simulink model "pendulum_2"  (R2023b)
settings: Solver=VariableStepAuto  StartTime=0.0  StopTime=5  RelTol=1e-3
values from neighbouring files (symbols this model uses):
  A = [0   1 ... (first row only)    [DC_motor_example_LQR_v2.m]    (also in inverted_pendulum_main.m = [ 0         0               1                   0)
  Ad = sysd.A    [inverted_pendulum_main.m]
  B = [0 ... (first row only)    [DC_motor_example_LQR_v2.m]    (also in inverted_pendulum_main.m = [       0)
  Bd = sysd.B    [inverted_pendulum_main.m]
  Cc = eye(4)    [inverted_pendulum_main.m]
  Cd = sysd.C    [inverted_pendulum_main.m]
  Dc = zeros(4, 1)    [inverted_pendulum_main.m]
  Dd = sysd.D    [inverted_pendulum_main.m]
  K = lqr(A,B,Q,R)    [DC_motor_example_LQR_v2.m]    (also in inverted_pendulum_main.m = lqr(sys, Qf, Rf))
  Kd = lqr(sysd, Qf, Rf)    [inverted_pendulum_main.m]
  Ts = 0.005    [inverted_pendulum_main.m]
  wc = pi    (= 3.14159265359)    [inverted_pendulum_main.m]
libraries: simulink x8
settings Model: Creator=loicdewit  LastModifiedBy=loicdewit

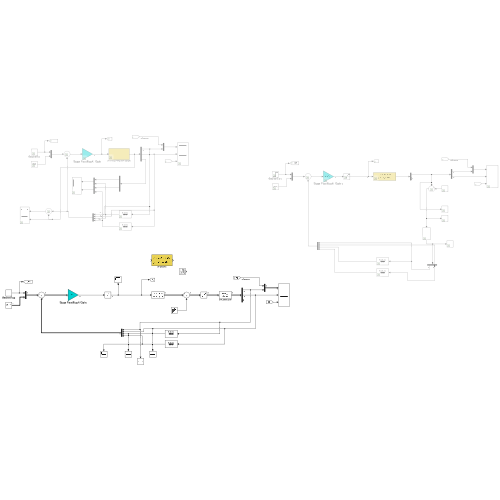
[thumbnail: Simulink's stored preview of the top-level diagram]
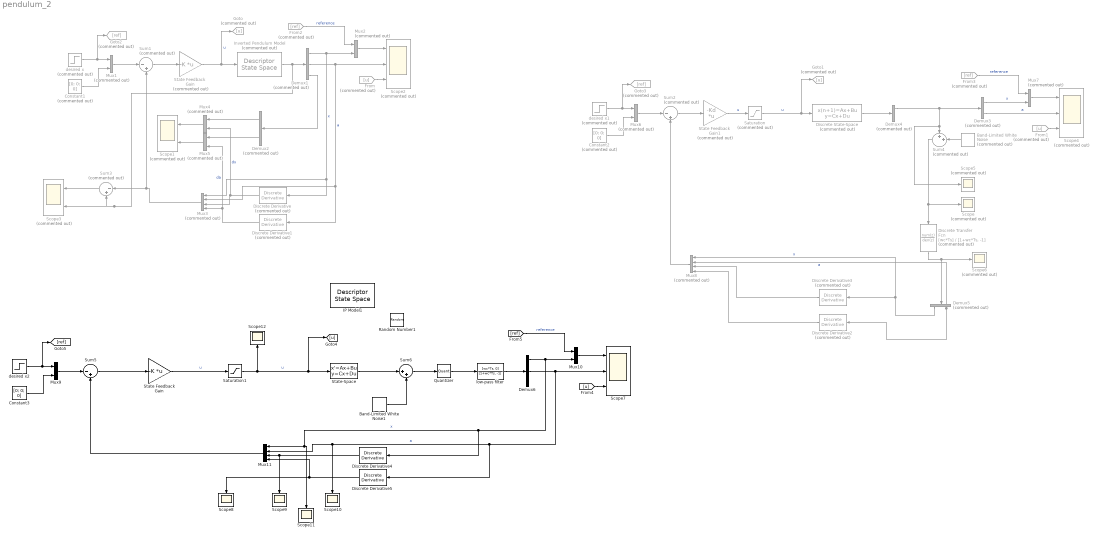
== system pendulum_2 ==
  Band-Limited White Noise : simulink/Sources/Band-Limited White Noise  Commented=on  Cov=[0.000001 * Ts]  Ts=Ts  seed=[13072002]  VectorParams1D=off
  Band-Limited White Noise1 : simulink/Sources/Band-Limited White Noise  Cov=[0.0001 * Ts]  Ts=Ts  seed=[13072002]  VectorParams1D=off
  Constant1 : Constant  Commented=on  Value=[0; 0; 0]
  Constant2 : Constant  Commented=on  Value=[0; 0; 0]
  Constant3 : Constant  Value=[0; 0; 0]  SampleTime=Ts
  Demux1 : Demux  Commented=on  Outputs=[1 1 2]
  Demux2 : Demux  Commented=on  Outputs=[1 1]
  Demux3 : Demux  Commented=on  Outputs=[1 1]
  Demux4 : Demux  Commented=on  Outputs=[2 2]
  Demux5 : Demux  Commented=on  Outputs=[1 1]
  Demux6 : Demux  Outputs=[1 1 2]
  Discrete Transfer Fcn : DiscreteTransferFcn  Commented=on  Numerator=[wc*Ts]  Denominator=[1+wc*Ts, -1]
  Discrete Derivative{,1..3} (4 alike) : simulink/Discrete/Discrete Derivative  Commented=on  gainval=1.0  ICPrevScaledInput=0.0  OutMin=[]  OutMax=[]  OutDataType=fixdt(1, 16)  OutScaling=2^-10  DoSatur=off
  Discrete Derivative4 : simulink/Discrete/Discrete Derivative  gainval=1.0  ICPrevScaledInput=0.0  OutMin=[]  OutMax=[]  OutDataType=fixdt(1, 16)  OutScaling=2^-10  DoSatur=off
  Discrete Derivative5 : simulink/Discrete/Discrete Derivative  gainval=1.0  ICPrevScaledInput=0.0  OutMin=[]  OutMax=[]  OutDataType=fixdt(1, 16)  OutScaling=2^-10  DoSatur=off
  Discrete State-Space : DiscreteStateSpace  Commented=on  A=Ad  B=Bd  C=Cd  D=Dd  SampleTime=Ts
  From : From  Commented=on  GotoTag=u
  From1 : From  Commented=on  GotoTag=u
  From2 : From  Commented=on  GotoTag=ref
  From3 : From  Commented=on  GotoTag=ref
  Goto : Goto  Commented=on  GotoTag=u
  Goto1 : Goto  Commented=on  GotoTag=u
  Goto2 : Goto  Commented=on  GotoTag=ref
  Goto3 : Goto  Commented=on  GotoTag=ref
  IP Model1 : DescriptorStateSpace  E=eye(4)  A=A  B=B  C=Cc  D=Dc
  Inverted Pendulum Model : DescriptorStateSpace  Commented=on  E=eye(4)  A=A  B=B  C=Cc  D=Dc
  Mux{1..2,4..7} (6 alike) : Mux  Commented=on  Inputs=2
  Mux10 : Mux  Inputs=2
  Mux11 : Mux
  Mux3 : Mux  Commented=on
  Mux8 : Mux  Commented=on
  Mux9 : Mux  Inputs=2
  Quantizer : Quantizer  QuantizationInterval=20/(2^16)
  Random Number1 : RandomNumber  Variance=1e-3  SampleTime=Ts
  Saturation : Saturate  Commented=on  UpperLimit=5  LowerLimit=-5
  Saturation1 : Saturate  UpperLimit=5  LowerLimit=-5
  Scope : Scope  Commented=on
  Scope1 : Scope  Commented=on  NumInputPorts=2
  Scope{8..12} (5 alike) : Scope
  Scope2 : Scope  Commented=on  NumInputPorts=3
  Scope3 : Scope  Commented=on  NumInputPorts=2
  Scope4 : Scope  Commented=on  NumInputPorts=3
  Scope5 : Scope  Commented=on
  Scope6 : Scope  Commented=on
  Scope7 : Scope  NumInputPorts=3
  State Feedback  Gain : Gain  Commented=on  Gain=-K  Multiplication=Matrix(K*u)
  State Feedback  Gain1 : Gain  Commented=on  Gain=-Kd  Multiplication=Matrix(K*u)
  State Feedback Gain : Gain  Gain=-K  Multiplication=Matrix(K*u)
  State-Space : StateSpace  A=A  B=B  C=Cc  D=Dc  InitialCondition=0
  Sum1 : Sum  Commented=on  Inputs=|-+
  Sum2 : Sum  Commented=on  Inputs=|-+
  Sum3 : Sum  Commented=on  Inputs=|-+
  Sum4 : Sum  Commented=on  Inputs=++|
  Sum5 : Sum  Inputs=|-+
  Sum6 : Sum  Inputs=|++
  desired x : Step  Commented=on  After=0.1  SampleTime=0
  desired x1 : Step  Commented=on  After=0.1  SampleTime=0
  desired x2 : Step  After=0  SampleTime=Ts
  low-pass filter : DiscreteTransferFcn  Numerator=[wc*Ts, 0]  Denominator=[1+wc*Ts, -1]
  wires:
  Sum1/1 -> State Feedback  Gain/1
  Mux2/1 -> Scope2/1
  Mux1/1 -> Sum1/1
  Demux1/1 -> Discrete Derivative/1, Mux3/1, Mux2/2  "x"
  From2/1 -> Mux2/1  "reference"
  From/1 -> Scope2/3
  State Feedback  Gain/1 -> Goto/1, Inverted Pendulum Model/1  "u"
  Demux1/2 -> Discrete Derivative1/1, Mux3/2, Scope2/2  "a"
  desired x/1 -> Goto2/1, Mux1/1
  Constant1/1 -> Mux1/2
  Inverted Pendulum Model/1 -> Scope3/2, Sum3/2, Demux1/1
  Discrete Derivative1/1 -> Mux5/2, Mux3/4  "da"
  Discrete Derivative/1 -> Mux4/2, Mux3/3  "dx"
  Demux1/3 -> Demux2/1
  Demux2/1 -> Mux4/1
  Mux4/1 -> Scope1/1
  Demux2/2 -> Mux5/1
  Mux5/1 -> Scope1/2
  Mux3/1 -> Sum1/2, Sum3/1
  Sum3/1 -> Scope3/1
  Demux3/2 -> Scope4/2  "a"
  Mux6/1 -> Sum2/1
  Constant2/1 -> Mux6/2
  desired x1/1 -> Goto3/1, Mux6/1
  From1/1 -> Scope4/3
  Sum2/1 -> State Feedback  Gain1/1
  Saturation/1 -> Discrete State-Space/1, Goto1/1  "u"
  Discrete State-Space/1 -> Demux4/1
  Mux7/1 -> Scope4/1
  Demux3/1 -> Mux7/2  "x"
  From3/1 -> Mux7/1  "reference"
  Discrete Derivative3/1 -> Mux8/3
  Discrete Derivative2/1 -> Mux8/4
  Mux8/1 -> Sum2/2
  Demux4/1 -> Scope5/1, Sum4/1, Demux3/1
  Band-Limited White Noise/1 -> Sum4/2
  Sum4/1 -> Discrete Transfer Fcn/1, Scope/1
  Discrete Transfer Fcn/1 -> Demux5/1, Scope6/1
  Demux5/1 -> Discrete Derivative3/1, Mux8/1  "x"
  Demux5/2 -> Discrete Derivative2/1, Mux8/2  "a"
  State Feedback  Gain1/1 -> Saturation/1  "u"
  Demux6/2 -> Mux11/2, Scope10/1, Discrete Derivative5/1, Scope7/2  "a"
  Mux9/1 -> Sum5/1
  Constant3/1 -> Mux9/2
  desired x2/1 -> [ref], Mux9/1
  [u] -> Scope7/3
  Sum5/1 -> State Feedback Gain/1
  Mux10/1 -> Scope7/1
  Demux6/1 -> Scope11/1, Mux11/1, Discrete Derivative4/1, Mux10/2  "x"
  [ref] -> Mux10/1  "reference"
  Sum6/1 -> Quantizer/1
  Discrete Derivative5/1 -> Scope8/1, Mux11/4
  Discrete Derivative4/1 -> Scope9/1, Mux11/3
  Mux11/1 -> Sum5/2
  State Feedback Gain/1 -> Saturation1/1  "u"
  Saturation1/1 -> Scope12/1, State-Space/1, [u]  "u"
  Band-Limited White Noise1/1 -> Sum6/2
  Quantizer/1 -> low-pass filter/1
  low-pass filter/1 -> Demux6/1
  State-Space/1 -> Sum6/1
